simulink model "q1"  (R2021b)
settings: Solver=VariableStepAuto  StartTime=0.0  StopTime=100.0  RelTol=1e-3
libraries: simulink x1
settings Model: Creator=ASUS  LastModifiedBy=ASUS

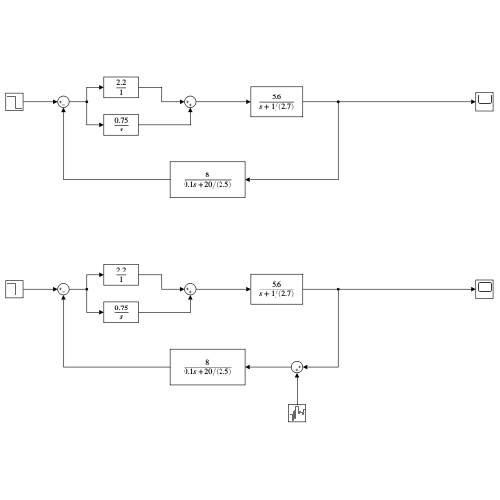
[thumbnail: Simulink's stored preview of the top-level diagram]
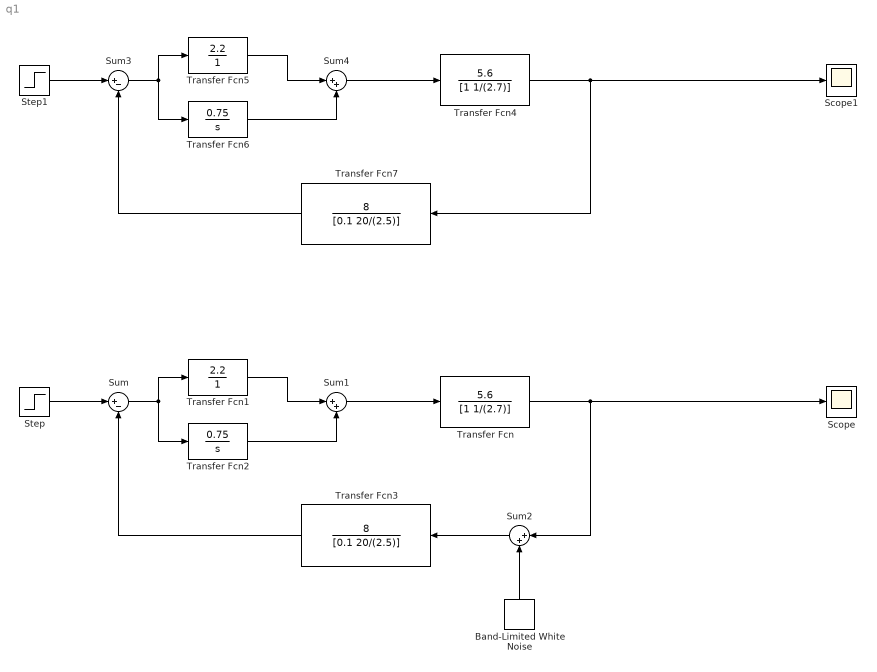
== system q1 ==
  Band-Limited White Noise : simulink/Sources/Band-Limited White Noise  Cov=[0.01]  Ts=0.001  seed=[23341]
  Scope : Scope
  Scope1 : Scope
  Step : Step  Time=0  Before=10  SampleTime=0
  Step1 : Step  Time=0  Before=10  SampleTime=0
  Sum : Sum  Inputs=|+-
  Sum1 : Sum  Inputs=|++
  Sum2 : Sum  Inputs=|++
  Sum3 : Sum  Inputs=|+-
  Sum4 : Sum  Inputs=|++
  Transfer Fcn : TransferFcn  Numerator=[5.6]  Denominator=[1 1/(2.7)]
  Transfer Fcn1 : TransferFcn  Numerator=[2.2]  Denominator=[1]
  Transfer Fcn2 : TransferFcn  Numerator=[0.75]  Denominator=[1 0]
  Transfer Fcn3 : TransferFcn  Numerator=[8]  Denominator=[0.1 20/(2.5)]
  Transfer Fcn4 : TransferFcn  Numerator=[5.6]  Denominator=[1 1/(2.7)]
  Transfer Fcn5 : TransferFcn  Numerator=[2.2]  Denominator=[1]
  Transfer Fcn6 : TransferFcn  Numerator=[0.75]  Denominator=[1 0]
  Transfer Fcn7 : TransferFcn  Numerator=[8]  Denominator=[0.1 20/(2.5)]
  wires:
  Step/1 -> Sum/1
  Sum/1 -> Transfer Fcn2/1, Transfer Fcn1/1
  Transfer Fcn1/1 -> Sum1/1
  Transfer Fcn2/1 -> Sum1/2
  Sum1/1 -> Transfer Fcn/1
  Transfer Fcn/1 -> Sum2/1, Scope/1
  Transfer Fcn3/1 -> Sum/2
  Sum2/1 -> Transfer Fcn3/1
  Band-Limited White Noise/1 -> Sum2/2
  Transfer Fcn4/1 -> Transfer Fcn7/1, Scope1/1
  Sum4/1 -> Transfer Fcn4/1
  Transfer Fcn5/1 -> Sum4/1
  Transfer Fcn6/1 -> Sum4/2
  Sum3/1 -> Transfer Fcn6/1, Transfer Fcn5/1
  Transfer Fcn7/1 -> Sum3/2
  Step1/1 -> Sum3/1
